simulink model "GLO_tracking_model_no_ptu_dynamics_brett"  (R2017b)
settings: Solver=VariableStepAuto  StartTime=0.0  StopTime=117.2  MaxStep=0.01  RelTol=1e-4  EnableMultiTasking=on
libraries: dspstat3 x2, dspfdesign x1, simulink x1
settings Model: Creator=addiewan  LastModifiedBy=addiewan
settings DataIOCC: LimitDataPoints=on  SaveOutput=off  SaveTime=off
settings OptimizationCC: ExpressionDepthLimit=2147483647  LifeSpan=1
settings DebuggingCC: UnderspecifiedInitializationDetection=Classic  MergeDetectMultiDrivingBlocksExec=none  FcnCallInpInsideContextMsg=warning  AllowSymbolicDim=off  StateNameClashWarn=warning  SFUnexpectedBacktrackingDiag=warning  SFNoUnconditionalDefaultTransitionDiag=warning  SFExecutionAtInitializationDiag=none
settings CodeAppCC: StateflowObjectComments=on
settings GRTTargetCC: TargetLangStandard=C89/C90 (ANSI)  GeneratePreprocessorConditionals=Disable all  CombineOutputUpdateFcns=off  GRTInterface=on
settings ConfigComp: CovMetricSettings=dw  CovHtmlReporting=on  CovSaveCumulativeToWorkspaceVar=on  CovSaveSingleToWorkspaceVar=on  CovExternalEMLEnable=off

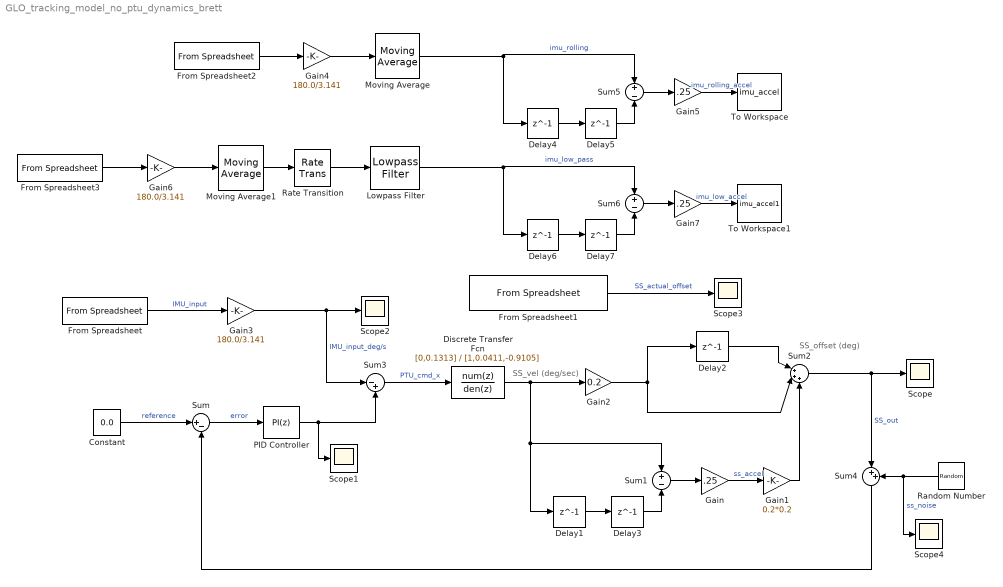
== system GLO_tracking_model_no_ptu_dynamics_brett ==
  note: SS_vel (deg/sec)
  note: SS_offset (deg)
  Constant : Constant  Value=0.0
  Delay{1..7} (7 alike) : Delay  DelayLength=1  InitialCondition=0.523
  Discrete Transfer Fcn : DiscreteTransferFcn  Numerator=[0,0.1313]  Denominator=[1,0.0411,-0.9105]
  From Spreadsheet : FromSpreadsheet  FileName=C:\git_repos\GLO_Tracking\testing\Simulation\IMU_forSumulink.xlsx  SampleTime=-1
  From Spreadsheet1 : FromSpreadsheet  FileName=C:\git_repos\GLO_Tracking\testing\Simulation\SS_output_RUN6_20180710.xlsx  SampleTime=-1
  From Spreadsheet2 : FromSpreadsheet  FileName=C:\git_repos\GLO_Tracking\testing\Simulation\IMU_forSumulink.xlsx
  From Spreadsheet3 : FromSpreadsheet  FileName=C:\git_repos\GLO_Tracking\testing\Simulation\IMU_forSumulink.xlsx  SampleTime=-1
  Gain : Gain  Gain=.25
  Gain1 : Gain  Gain=0.2*0.2
  Gain2 : Gain  Gain=0.2
  Gain3 : Gain  Gain=180.0/3.141
  Gain4 : Gain  Gain=180.0/3.141
  Gain5 : Gain  Gain=.25
  Gain6 : Gain  Gain=180.0/3.141
  Gain7 : Gain  Gain=.25
  Lowpass Filter : dspfdesign/Lowpass Filter  FilterType=FIR  DesignForMinimumOrder=on  FilterOrder=50  PassbandFrequency=1e-6  StopbandFrequency=4e-2  PassbandRipple=0.1  StopbandAttenuation=80  InheritSampleRate=off  SampleRate=5  SimulateUsing=Interpreted execution  roundingMode=Floor  coeffsDataTypeStr=fixdt(1,16)
  Moving Average : dspstat3/Moving Average  Method=Sliding window  SpecifyWindowLength=on  WindowLength=400  ForgettingFactor=0.9  SimulateUsing=Code generation
  Moving Average1 : dspstat3/Moving Average  Method=Sliding window  SpecifyWindowLength=on  WindowLength=400  ForgettingFactor=0.9  SimulateUsing=Code generation
  PID Controller : simulink/Continuous/PID Controller  Controller=PI  TimeDomain=Discrete-time  SampleTime=.2  IntegratorMethod=Trapezoidal  FilterMethod=Trapezoidal  Form=Parallel  UseFilter=off  ControllerParametersSource=internal  P=21.6830216072567  I=0  D=3.35511074926597  N=1.62461583533884  InitialConditionSource=internal  InitialConditionForIntegrator=0  InitialConditionForFilter=0  ExternalReset=none  LimitOutput=off  UpperSaturationLimit=inf  LowerSaturationLimit=-inf  LinearizeAsGain=on  AntiWindupMode=none  Kb=1  TrackingMode=off  Kt=1  PParamMin=[]  PParamMax=[]  IParamMin=[]  IParamMax=[]  DParamMin=[]  DParamMax=[]  NParamMin=[]  NParamMax=[]  KbParamMin=[]  KbParamMax=[]  KtParamMin=[]  KtParamMax=[]  POutMin=[]  POutMax=[]  IOutMin=[]  IOutMax=[]  DOutMin=[]  DOutMax=[]  NOutMin=[]  NOutMax=[]  KbOutMin=[]  KbOutMax=[]  KtOutMin=[]  KtOutMax=[]  IntegratorOutMin=[]  IntegratorOutMax=[]  FilterOutMin=[]  FilterOutMax=[]  SumOutMin=[]  SumOutMax=[]  SumI1OutMin=[]  SumI1OutMax=[]  SumI2OutMin=[]  SumI2OutMax=[]  SumI3OutMin=[]  SumI3OutMax=[]  SumDOutMin=[]  SumDOutMax=[]  SaturationOutMin=[]  SaturationOutMax=[]  IntegratorContinuousStateAttributes=''  IntegratorStateMustResolveToSignalObject=off  IntegratorRTWStateStorageClass=Auto  FilterContinuousStateAttributes=''  FilterStateMustResolveToSignalObject=off  FilterRTWStateStorageClass=Auto  DifferentiatorICPrevScaledInput=0  DifferentiatorOutMin=[]  DifferentiatorOutMax=[]  InitialConditionSetting=State (most efficient)  FilterDiffOutCoefMin=[]  FilterDiffOutCoefMax=[]  SumDenOutMin=[]  SumDenOutMax=[]  SumNumOutMin=[]  SumNumOutMax=[]  ReciprocalOutMin=[]  ReciprocalOutMax=[]  DivideOutMin=[]  DivideOutMax=[]  TunerSelectOption=Transfer Function Based (PID Tuner App)
  Random Number : RandomNumber  Variance=(.005*0.005)/sqrt(10)  SampleTime=1
  Rate Transition : RateTransition  OutPortSampleTimeOpt=Inherit
  Scope{,1..4} (5 alike) : Scope
  Sum : Sum  Inputs=|+-
  Sum1 : Sum  Inputs=+-
  Sum2 : Sum  Inputs=|+++
  Sum3 : Sum  Inputs=|-+
  Sum4 : Sum  Inputs=|++
  Sum5 : Sum  Inputs=+-
  Sum6 : Sum  Inputs=+-
  To Workspace : ToWorkspace  VariableName=imu_accel  SampleTime=-1
      settings: Save2DSignal=2-D array (concatenate along first dimension)
  To Workspace1 : ToWorkspace  VariableName=imu_accel1  SampleTime=-1
      settings: Save2DSignal=2-D array (concatenate along first dimension)
  wires:
  Constant/1 -> Sum/1  "reference"
  Sum1/1 -> Gain/1
  Gain/1 -> Gain1/1  "ss_accel"
  Gain1/1 -> Sum2/3
  Delay2/1 -> Sum2/1
  Sum2/1 -> Scope/1, Sum4/1  "SS_out"
  Gain2/1 -> Delay2/1, Sum2/2
  Sum/1 -> PID Controller/1  "error"
  PID Controller/1 -> Scope1/1, Sum3/2
  From Spreadsheet1/1 -> Scope3/1  "SS_actual_offset"
  From Spreadsheet/1 -> Gain3/1  "IMU_input"
  Delay1/1 -> Delay3/1
  Delay3/1 -> Sum1/2
  Sum3/1 -> Discrete Transfer Fcn/1  "PTU_cmd_x"
  Sum4/1 -> Sum/2
  Random Number/1 -> Scope4/1, Sum4/2  "ss_noise"
  Discrete Transfer Fcn/1 -> Gain2/1, Delay1/1, Sum1/1
  Gain3/1 -> Sum3/1, Scope2/1  "IMU_input_deg/s"
  From Spreadsheet2/1 -> Gain4/1
  Gain4/1 -> Moving Average/1
  Moving Average/1 -> Sum5/1, Delay4/1  "imu_rolling"
  Sum5/1 -> Gain5/1
  Delay5/1 -> Sum5/2
  Delay4/1 -> Delay5/1
  Gain5/1 -> To Workspace/1  "imu_rolling_accel"
  Delay7/1 -> Sum6/2
  Gain7/1 -> To Workspace1/1  "imu_low_accel"
  Sum6/1 -> Gain7/1
  Lowpass Filter/1 -> Sum6/1, Delay6/1  "imu_low_pass"
  Delay6/1 -> Delay7/1
  From Spreadsheet3/1 -> Gain6/1
  Rate Transition/1 -> Lowpass Filter/1
  Gain6/1 -> Moving Average1/1
  Moving Average1/1 -> Rate Transition/1
